simulink model "model_response"  (R2024a)
settings: Solver=VariableStepAuto  StartTime=0.0  StopTime=10  RelTol=1e-3
undefined symbols (not defined in the file): A, B, C, F, K, u_amp, u_w, useSine
libraries: simulink_extras x2
settings Model: Creator=carso  LastModifiedBy=dunni

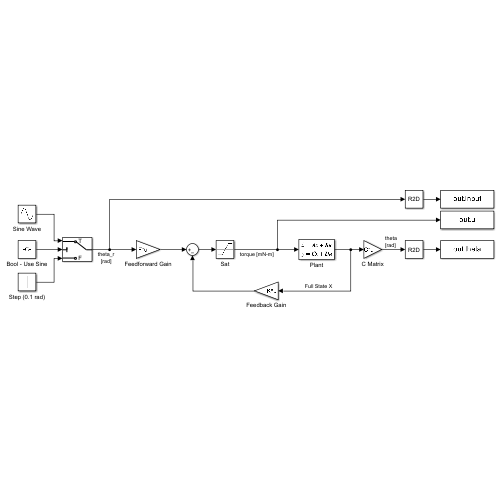
[thumbnail: Simulink's stored preview of the top-level diagram]
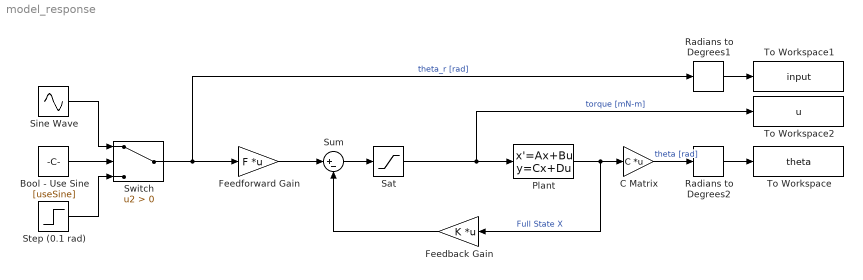
== system model_response ==
  Bool - Use Sine : Constant  Value=[useSine]
  C Matrix : Gain  Gain=C  Multiplication=Matrix(K*u)
  Feedback Gain : Gain  Gain=K  Multiplication=Matrix(K*u)
  Feedforward Gain : Gain  Gain=F  Multiplication=Matrix(K*u)
  Plant : StateSpace  A=A  B=B  C=eye(4)  D=zeros(4,1)  InitialCondition=0
  Radians to Degrees1 : simulink_extras/Transformations/Radians to Degrees
  Radians to Degrees2 : simulink_extras/Transformations/Radians to Degrees
  Sat : Saturate  UpperLimit=67  LowerLimit=-67
  Sine Wave : Sin  Amplitude=[u_amp]  Frequency=[u_w]  SampleTime=0
  Step (0.1 rad) : Step  After=0.1  SampleTime=0
  Sum : Sum  Inputs=|+-
  Switch : Switch  Criteria=u2 > Threshold  SaturateOnIntegerOverflow=off  InputSameDT=off
  To Workspace : ToWorkspace  VariableName=theta  SaveFormat=Timeseries  SampleTime=-1
  To Workspace1 : ToWorkspace  VariableName=input  SaveFormat=Timeseries  SampleTime=-1
  To Workspace2 : ToWorkspace  VariableName=u  SaveFormat=Timeseries  SampleTime=-1
  wires:
  Sum/1 -> Sat/1
  Switch/1 -> Radians to Degrees1/1, Feedforward Gain/1  "theta_r [rad]"
  Bool - Use Sine/1 -> Switch/2
  Step (0.1 rad)/1 -> Switch/3
  Sine Wave/1 -> Switch/1
  Sat/1 -> To Workspace2/1, Plant/1  "torque [mN-m]"
  Feedback Gain/1 -> Sum/2
  Plant/1 -> C Matrix/1, Feedback Gain/1  "Full State X"
  Feedforward Gain/1 -> Sum/1
  C Matrix/1 -> Radians to Degrees2/1  "theta [rad]"
  Radians to Degrees1/1 -> To Workspace1/1
  Radians to Degrees2/1 -> To Workspace/1
